simulink model "PD"  (R2018a)
settings: Solver=FixedStepAuto  StartTime=0.0  StopTime=7  FixedStep=0.01  RelTol=1e-3  EnableMultiTasking=on
libraries: simulink x1
settings Model: Creator=hoang  LastModifiedBy=phamn
settings DataIOCC: LimitDataPoints=on
settings OptimizationCC: LifeSpan=inf
settings DebuggingCC: AllowSymbolicDim=off  SFUnexpectedBacktrackingDiag=warning  SFNoUnconditionalDefaultTransitionDiag=warning  SFExecutionAtInitializationDiag=none
settings ModelReferenceCC: PropagateSignalLabelsOutOfModel=off
settings CodeAppCC: StateflowObjectComments=on
settings GRTTargetCC: TargetLangStandard=C89/C90 (ANSI)
settings ConfigComp: CovMetricSettings=dw  CovHtmlReporting=on  CovSaveCumulativeToWorkspaceVar=on  CovSaveSingleToWorkspaceVar=on  CovExternalEMLEnable=off

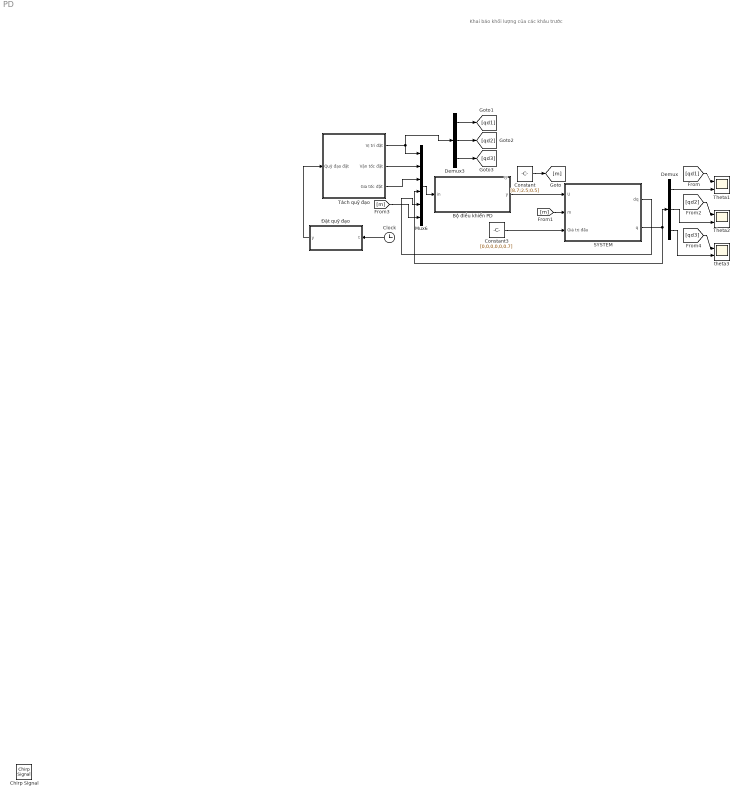
== system PD ==
  note: Khai báo khối lượng của các khâu trước
  note: U
  Bộ điều khiển PD : MATLAB Function  TreatAsAtomicUnit=on
  Clock : Clock
      settings: Decimation=100
  Constant : Constant  Value=[8.7;2.5;0.5]
  Constant3 : Constant  Value=[0,0,0,0,0,0.7]
  Demux : Demux  Outputs=3
  Demux3 : Demux  Outputs=3
  Mux6 : Mux  Inputs=6
  "SYSTEM " : Subsystem
  Theta1 : Scope  NumInputPorts=2
  Theta2 : Scope  NumInputPorts=2
  Tách quỹ đạo : Subsystem
  theta3 : Scope  NumInputPorts=2
  Đặt quỹ đạo : MATLAB Function  TreatAsAtomicUnit=on
  Chirp Signal : simulink/Sources/Chirp Signal  IOType=siggen  f1=0.1  T=100  f2=1
  wires:
  Constant/1 -> [m]
  "SYSTEM "/1(dq) -> Mux6/5
  "SYSTEM "/2(q) -> Mux6/4, Demux/1
  Mux6/1 -> Bộ điều khiển PD/1(in)
  [m] -> Mux6/6
  Clock/1 -> Đặt quỹ đạo/1(t)
  Tách quỹ đạo/2(Vận tốc đặt) -> Mux6/2
  Tách quỹ đạo/3(Gia tốc đặt) -> Mux6/3
  Demux/2 -> Theta2/2
  Demux/3 -> theta3/2
  Demux3/1 -> [qd1]
  Demux3/3 -> [qd3]
  Demux3/2 -> [qd2]
  Tách quỹ đạo/1(Vị trí đặt) -> Demux3/1, Mux6/1
  [qd1] -> Theta1/1
  [qd2] -> Theta2/1
  [qd3] -> theta3/1
  Bộ điều khiển PD/1(y) -> "SYSTEM "/1(U)
  [m] -> "SYSTEM "/2(m)
  Constant3/1 -> "SYSTEM "/3(Giá trị đầu)
  Demux/1 -> Theta1/2
  Đặt quỹ đạo/1(y) -> Tách quỹ đạo/1(Quỹ đạo đặt)

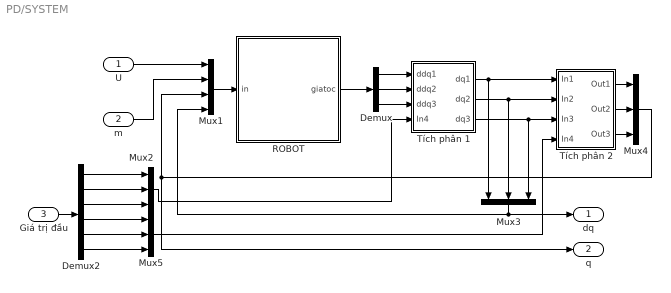
== system PD/SYSTEM  ==
  U : Inport
  m : Inport  Port=2
  Giá trị đầu : Inport  Port=3
  Demux : Demux  Outputs=3
  Demux2 : Demux  Outputs=6
  Mux1 : Mux
  Mux{2..5} (4 alike) : Mux  Inputs=3
  ROBOT : MATLAB Function  TreatAsAtomicUnit=on
  Tích phân 1 : Subsystem
  Tích phân 2 : Subsystem
  dq : Outport
  q : Outport  Port=2
  wires:
  ROBOT/1(giatoc) -> Demux/1
  Giá trị đầu/1 -> Demux2/1
  Mux3/1 -> Mux1/4, dq/1
  m/1 -> Mux1/2
  Mux4/1 -> q/1, Mux1/3
  Mux1/1 -> ROBOT/1(in)
  U/1 -> Mux1/1
  Demux2/3 -> Mux2/3
  Demux2/2 -> Mux2/2
  Demux2/1 -> Mux2/1
  Demux2/5 -> Mux5/2
  Demux2/6 -> Mux5/3
  Demux2/4 -> Mux5/1
  Tích phân 1/2(dq2) -> Tích phân 2/2(In2), Mux3/2
  Tích phân 1/3(dq3) -> Tích phân 2/3(In3), Mux3/3
  Tích phân 1/1(dq1) -> Tích phân 2/1(In1), Mux3/1
  Demux/1 -> Tích phân 1/1(ddq1)
  Demux/2 -> Tích phân 1/2(ddq2)
  Demux/3 -> Tích phân 1/3(ddq3)
  Mux2/1 -> Tích phân 1/4(In4)
  Mux5/1 -> Tích phân 2/4(In4)
  Tích phân 2/1(Out1) -> Mux4/1
  Tích phân 2/2(Out2) -> Mux4/2
  Tích phân 2/3(Out3) -> Mux4/3

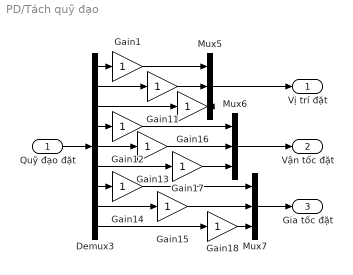
== system PD/Tách quỹ đạo ==
  Quỹ đạo đặt : Inport
  Demux3 : Demux  Outputs=9
  Gain{1,11..18} (9 alike) : Gain
  Mux5 : Mux  Inputs=3
  Mux6 : Mux  Inputs=3
  Mux7 : Mux  Inputs=3
  Vị trí đặt : Outport
  Vận tốc đặt : Outport  Port=2
  Gia tốc đặt : Outport  Port=3
  wires:
  Demux3/8 -> Gain15/1
  Demux3/9 -> Gain18/1
  Demux3/6 -> Gain17/1
  Gain11/1 -> Mux5/2
  Gain12/1 -> Mux6/1
  Gain13/1 -> Mux6/2
  Gain18/1 -> Mux7/3
  Gain1/1 -> Mux5/1
  Mux5/1 -> Vị trí đặt/1
  Demux3/3 -> Gain16/1
  Gain17/1 -> Mux6/3
  Demux3/7 -> Gain14/1
  Mux6/1 -> Vận tốc đặt/1
  Gain16/1 -> Mux5/3
  Demux3/2 -> Gain11/1
  Gain14/1 -> Mux7/1
  Demux3/1 -> Gain1/1
  Gain15/1 -> Mux7/2
  Mux7/1 -> Gia tốc đặt/1
  Quỹ đạo đặt/1 -> Demux3/1
  Demux3/4 -> Gain12/1
  Demux3/5 -> Gain13/1

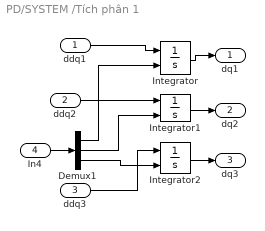
== system PD/SYSTEM /Tích phân 1 ==
  ddq1 : Inport
  ddq2 : Inport  Port=2
  ddq3 : Inport  Port=3
  In4 : Inport  Port=4
  Demux1 : Demux  Outputs=3
  Integrator : Integrator  InitialConditionSource=external
  Integrator1 : Integrator  InitialConditionSource=external
  Integrator2 : Integrator  InitialConditionSource=external
  dq1 : Outport
  dq2 : Outport  Port=2
  dq3 : Outport  Port=3
  wires:
  Demux1/2 -> Integrator1/2
  In4/1 -> Demux1/1
  Demux1/1 -> Integrator/2
  Demux1/3 -> Integrator2/2
  ddq3/1 -> Integrator2/1
  ddq2/1 -> Integrator1/1
  Integrator2/1 -> dq3/1
  ddq1/1 -> Integrator/1
  Integrator/1 -> dq1/1
  Integrator1/1 -> dq2/1

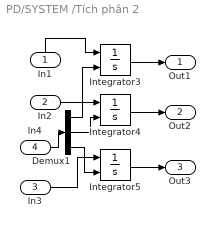
== system PD/SYSTEM /Tích phân 2 ==
  In1 : Inport
  In2 : Inport  Port=2
  In3 : Inport  Port=3
  In4 : Inport  Port=4
  Demux1 : Demux  Outputs=3
  Integrator3 : Integrator  InitialConditionSource=external
  Integrator4 : Integrator  InitialConditionSource=external
  Integrator5 : Integrator  InitialConditionSource=external
  Out1 : Outport
  Out2 : Outport  Port=2
  Out3 : Outport  Port=3
  wires:
  In4/1 -> Demux1/1
  Demux1/1 -> Integrator3/2
  Demux1/2 -> Integrator4/2
  In2/1 -> Integrator4/1
  In3/1 -> Integrator5/1
  In1/1 -> Integrator3/1
  Demux1/3 -> Integrator5/2
  Integrator3/1 -> Out1/1
  Integrator4/1 -> Out2/1
  Integrator5/1 -> Out3/1

== matlab function PD/Đặt quỹ đạo ==
  data: t input; y output
function y = Quy_dao(t)
%gioi han tung khop
qd1 = (2*pi/3)*sin(t/4);
qd2 = (pi/2)*sin(t/4);
qd3 = (3*pi/4)*sin(t/4);

vd1 = (pi/6)*cos(t/4);
vd2 = (pi/8)*cos(t/4);
vd3 = (3*pi/16)*cos(t/4);

ad1 = (-pi/24)*sin(t/4);
ad2 = (-pi/32)*sin(t/4);
ad3 = (-3*pi/64)*sin(t/4);

daura = [qd1;qd2;qd3;vd1;vd2;vd3;ad1;ad2;ad3];
y = daura;
end

== matlab function PD/Bộ điều khiển PD ==
  data: in input; y output
function y = dieukhien(in)
%#codegen:
% Dau vao: 
QD = in(1:3); VD = in(4:6);AD = in(7:9); Q = in(10:12); V = in(13:15);
qd1  =QD(1); qd2  = QD(2); qd3 = QD(3) ; vd1 = VD(1); vd2 = VD(2); vd3 = VD(3);
ad1 = AD(1); ad2 = AD(2); ad3 = AD(3);MV = in(16:18);
q1 = Q(1); q2 = Q(2); q3 = Q(3); dq1 = V(1); dq2 = V(2); dq3 = V(3);
qd = [qd1;qd2;qd3]; vd = [vd1;vd2;vd3]; ad = [ad1;ad2;ad3];
q = [q1;q2;q3]; v = [dq1;dq2;dq3];
% Khai bao cac dai luong 
a1 = 1.25; a2 = 1.25; a3 = 0.75; l1 = a1/2; l2 = a2/2; l3 = a3/2; % DV : m
m1 = 336.08 ; m2 = 217.55; m3 = 73.49 ; % DV kg
I1z = 0.1092; I2z = 0.4813; I3z = 0.0642;g = 9.81;

kp = diag([2500 2500 2500]); kd = diag([100 100 100]);

e = kp*(qd-q)+kd*(vd-v);
Avao  = ad+e;
% Khai bao cac ma tran 
%Ma tran khoi luong
m11 = m1*(a1-l1)^2+m2*((a2-l2)^2+2*a1*a2*cos(q2)-2*a1*l2*cos(q2)+a1^2)+m3*(2*a1*a2*cos(q2)+a1^2+a2^2+a3^2+l3^2-2*a3*l3+2*(a3-l3)*(a1*cos(q2+q3)+a2*cos(q3)))+I1z+I2z+I3z;
m12 = m2*((a2-l2)^2+a1*cos(q2)*(a2-l2))+m3*(a2^2+a3^2+l3^2+(a3-l3)*(a1*cos(q2+q3)-2*a2*cos(q3))+a1*a2*cos(q2)-2*a3*l3)+I2z+I3z;
m13 = m3*(a3^2+l3^2+(a3-l3)*(a1*cos(q2+q3)+a2*cos(q3))-2*a3*l3)+I3z;
m21 = m12;
m22 = m2*(a2-l2)^2+m3*(a2^2+2*a2*(a3-l3)*cos(q3)+(a3-l3)^2)+I2z+I3z;
m23 = m3*(a2*(a3-l3)*cos(q3)+(a3-l3)^2)+I3z;
m31 = m13;
m32 = m23;
m33 = m3*(a3-l3)^2+I3z;

M = [m11 m12 m13; m21 m22 m23; m31 m32 m33];

%Ma tran collioris: 

c11 = ((-2*a1*m2*sin(q2)*(a2-l2))+(2*a1*(a3-l3)*sin(q2+q3)-2*a1*a2*sin(q2)*m3))*dq2+((-2*a1*sin(q2+q3)*(a3-l3))-2*sin(q3)*a2*(a3-l3))*m3*dq3;
c12 = (-a1*sin(q2)*(a2-l2)*m2+(-a1*sin(q2+q3)*(a3-l3)-a1*a2*sin(q2))*m3)*dq2+(-a1*sin(q2+q3)*(a3-l3)-2*sin(q3)*a2*(a3-l3))*m3*dq3;
c13 = -m3*a1*sin(q2+q3)*(a3-l3)*dq2-(a3-l3)*m3*(a1*sin(q2+q3)+a2*sin(q3))*dq3;
c21 = (a1*sin(q2)*m2*(a2-l2)+(-a1*sin(q2+q3)*(l2-a3)+a1*a2*sin(q2))*m3)*dq1+(-0.5*a1*sin(q2)*m2*(a2-l2)+(0.5*a1*sin(q2+q3)*(l3-a3)-0.5*a1*a2*sin(q2))*m3)*dq2+(0.5*a1*sin(q2+q3)*(l3-a3)+2*sin(q3)*a2*(l3-a3))*m3*dq3;
c22 = (0.5*a1*sin(q2)*(a2-l2)*m2-(0.5*a1*sin(q2+q3)*(a3-l3)+0.5*a1*a2*sin(q2))*m3)*dq1-2*m3*sin(q3)*a2*(a3-l3)*dq3;
c23 = 0.5*m3*a1*sin(q2+q3)*(a3-l3)*dq1-m3*sin(q3)*a2*(a3-l3)*dq3;
c31 = (a1*sin(q2+q3)+sin(q3)*a2)*m3*(a3-l3)*dq1+(0.5*a1*sin(q2+q3)+a2*sin(q3))*(a3-l3)*m3*dq2+(0.5*a1*sin(q2+q3)-0.5*sin(q3)*a2)*(a3-l3)*m3*dq3;
c32 = (0.5*a1*sin(q2+q3)+a2*sin(q3))*(a3-l3)*m3*qd1+a2*sin(q3)*(a3-l3)*m3*dq2-0.5*a2*sin(q3)*(a3-l3)*m3*dq3;
c33 = 0.5*(a1*sin(q2+q3)+a2*sin(q3))*(a3-l3)*m3*dq1+0.5*a2*sin(q3)*(a3-l3)*m3*dq2;

C = [c11 c12 c13; c21 c22 c23; c31 c32 c33];

%Ma tran G: 

g1 = g*m1*a1*cos(q1)/2+g*(2*a1*cos(q1)+a2*cos(q1+q2))*m2/2+g*(2*a1*cos(q1)+a3*cos(q1+q2+q3)+2*a2*cos(q1+q2))*m3/2;
g2 = g*a2*m2*cos(q1+q2)/2+g*m3*(a3*cos(q1+q2+q3)+2*a2*cos(q1+q2))*m3/2;
g3 = g*a3*cos(q1+q2+q3)*m3/2;

G = [g1;g2;g3];

% Dau ra 
Uvao = M*Avao +C*v+G;

y = [Uvao];
end

== matlab function PD/SYSTEM /ROBOT ==
  data: in input; giatoc output
function giatoc = system(in)
%#codegen:
% Dau vao: 
UV= in(1:3); QV  = in(7:9); VV = in(10:12); MV = in(4:6);
q1  =QV(1); q2  = QV(2); q3 = QV(3) ; dq1 = VV(1); dq2 = VV(2); dq3 = VV(3);
u1  = UV(1); u2 = UV(2) ; u3 = UV(3);

% Khai bao cac dai luong 
a1 = 1.25; a2 = 1.25; a3 = 0.75; l1 = a1/2; l2 = a2/2; l3 = a3/2; % DV : m
% m1 = MV(1); m2 = MV(2); m3 = MV(3); % DV kg
m1 = 336.08 ; m2 = 217.55; m3 = 73.49
I1z = 0.1092; I2z = 0.4813; I3z = 0.0642;g = 9.81;

% Khai bao cac ma tran 
%Ma tran khoi luong
m11 = m1*(a1-l1)^2+m2*((a2-l2)^2+2*a1*a2*cos(q2)-2*a1*l2*cos(q2)+a1^2)+m3*(2*a1*a2*cos(q2)+a1^2+a2^2+a3^2+l3^2-2*a3*l3+2*(a3-l3)*(a1*cos(q2+q3)+a2*cos(q3)))+I1z+I2z+I3z;
m12 = m2*((a2-l2)^2+a1*cos(q2)*(a2-l2))+m3*(a2^2+a3^2+l3^2+(a3-l3)*(a1*cos(q2+q3)-2*a2*cos(q3))+a1*a2*cos(q2)-2*a3*l3)+I2z+I3z;
m13 = m3*(a3^2+l3^2+(a3-l3)*(a1*cos(q2+q3)+a2*cos(q3))-2*a3*l3)+I3z;
m21 = m12;
m22 = m2*(a2-l2)^2+m3*(a2^2+2*a2*(a3-l3)*cos(q3)+(a3-l3)^2)+I2z+I3z;
m23 = m3*(a2*(a3-l3)*cos(q3)+(a3-l3)^2)+I3z;
m31 = m13;
m32 = m23;
m33 = m3*(a3-l3)^2+I3z;

M = [m11 m12 m13; m21 m22 m23; m31 m32 m33];

%Ma tran collioris: 

c11 = ((-2*a1*m2*sin(q2)*(a2-l2))+(2*a1*(a3-l3)*sin(q2+q3)-2*a1*a2*sin(q2)*m3))*dq2+((-2*a1*sin(q2+q3)*(a3-l3))-2*sin(q3)*a2*(a3-l3))*m3*dq3;
c12 = (-a1*sin(q2)*(a2-l2)*m2+(-a1*sin(q2+q3)*(a3-l3)-a1*a2*sin(q2))*m3)*dq2+(-a1*sin(q2+q3)*(a3-l3)-2*sin(q3)*a2*(a3-l3))*m3*dq3;
c13 = -m3*a1*sin(q2+q3)*(a3-l3)*dq2-(a3-l3)*m3*(a1*sin(q2+q3)+a2*sin(q3))*dq3;
c21 = (a1*sin(q2)*m2*(a2-l2)+(-a1*sin(q2+q3)*(l2-a3)+a1*a2*sin(q2))*m3)*dq1+(-0.5*a1*sin(q2)*m2*(a2-l2)+(0.5*a1*sin(q2+q3)*(l3-a3)-0.5*a1*a2*sin(q2))*m3)*dq2+(0.5*a1*sin(q2+q3)*(l3-a3)+2*sin(q3)*a2*(l3-a3))*m3*dq3;
c22 = (0.5*a1*sin(q2)*(a2-l2)*m2-(0.5*a1*sin(q2+q3)*(a3-l3)+0.5*a1*a2*sin(q2))*m3)*dq1-2*m3*sin(q3)*a2*(a3-l3)*dq3;
c23 = 0.5*m3*a1*sin(q2+q3)*(a3-l3)*dq1-m3*sin(q3)*a2*(a3-l3)*dq3;
c31 = (a1*sin(q2+q3)+sin(q3)*a2)*m3*(a3-l3)*dq1+(0.5*a1*sin(q2+q3)+a2*sin(q3))*(a3-l3)*m3*dq2+(0.5*a1*sin(q2+q3)-0.5*sin(q3)*a2)*(a3-l3)*m3*dq3;
c32 = (0.5*a1*sin(q2+q3)+a2*sin(q3))*(a3-l3)*m3*dq1+a2*sin(q3)*(a3-l3)*m3*dq2-0.5*a2*sin(q3)*(a3-l3)*m3*dq3;
c33 = 0.5*(a1*sin(q2+q3)+a2*sin(q3))*(a3-l3)*m3*dq1+0.5*a2*sin(q3)*(a3-l3)*m3*dq2;

C = [c11 c12 c13; c21 c22 c23; c31 c32 c33];

%Ma tran G: 

g1 = g*m1*a1*cos(q1)/2+g*(2*a1*cos(q1)+a2*cos(q1+q2))*m2/2+g*(2*a1*cos(q1)+a3*cos(q1+q2+q3)+2*a2*cos(q1+q2))*m3/2;
g2 = g*a2*m2*cos(q1+q2)/2+g*m3*(a3*cos(q1+q2+q3)+2*a2*cos(q1+q2))*m3/2;
g3 = g*a3*cos(q1+q2+q3)*m3/2;

G = [g1;g2;g3];

% Dau ra 
U = [u1;u2;u3];
Qdot = [dq1;dq2;dq2];
Vdot = inv(M)*(U-G-C*Qdot);
giatoc = [Vdot];
end
